simulink model "mg467984"  (Simulink 7.2)
settings: Solver=ode45  StartTime=0.0  StopTime=10.0  RelTol=1e-3
libraries: simulink x2
settings Model: Creator=mtocci  LastModifiedBy=mtocci
settings OptimizationCC: InlineParams=on  EfficientMapNaN2IntZero=off
settings DebuggingCC: StrictBusMsg=ErrorOnBusTreatedAsVector

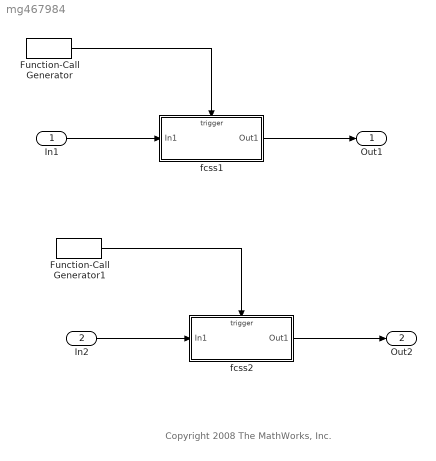
== system mg467984 ==
  note: Copyright 2008 The MathWorks, Inc.
  In1 : Inport  OutDataType=sfix(16)  OutScaling=2^0
  In2 : Inport  Port=2  OutDataType=sfix(16)  OutScaling=2^0
  Function-Call Generator : simulink/Ports & Subsystems/Function-Call Generator  sample_time=1  numberOfIterations=1
  Function-Call Generator1 : simulink/Ports & Subsystems/Function-Call Generator  sample_time=1  numberOfIterations=1
  fcss1 : Subsystem  TreatAsAtomicUnit=on
  fcss2 : Subsystem  TreatAsAtomicUnit=on
  Out1 : Outport  OutDataType=sfix(16)  OutScaling=2^0
  Out2 : Outport  Port=2  OutDataType=sfix(16)  OutScaling=2^0
  wires:
  Function-Call Generator/1 -> fcss1/Trigger
  In1/1 -> fcss1/1(In1)
  fcss1/1(Out1) -> Out1/1
  Function-Call Generator1/1 -> fcss2/Trigger
  In2/1 -> fcss2/1(In1)
  fcss2/1(Out1) -> Out2/1

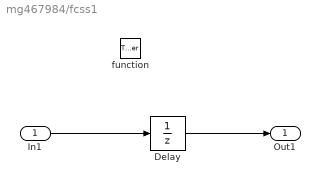
== system mg467984/fcss1 ==
  In1 : Inport  OutDataType=sfix(16)  OutScaling=2^0
  function : TriggerPort  TriggerType=function-call
  Delay : UnitDelay  X0=1  SampleTime=-1
  Out1 : Outport  OutDataType=sfix(16)  OutScaling=2^0
  wires:
  In1/1 -> Delay/1
  Delay/1 -> Out1/1

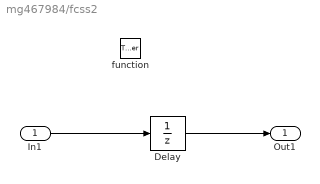
== system mg467984/fcss2 ==
  In1 : Inport  OutDataType=sfix(16)  OutScaling=2^0
  function : TriggerPort  TriggerType=function-call  SampleTimeType=periodic
  Delay : UnitDelay  X0=1  SampleTime=-1
  Out1 : Outport  OutDataType=sfix(16)  OutScaling=2^0
  wires:
  Delay/1 -> Out1/1
  In1/1 -> Delay/1
